simulink model "A_real_IGBT_Model"  (R2017b)
settings: Solver=ode23tb  StartTime=0.0  StopTime=0.01  MaxStep=1e-8  RelTol=1e-8  EnableMultiTasking=on
libraries: powerlib x12, powerlib_extras x2
Description:
  | Copyright 2008-2009 The MathWorks(TM), Inc.
settings Model: ExtModeTrigMode=oneshot  ExtModeArmWhenConnect=off  ExtModeAutoUpdateStatusClock=off  Creator=dkennedy  LastModifiedBy=Crazyyiwen
settings DataIOCC: SaveFormat=Array  SignalLoggingSaveFormat=ModelDataLogs  SignalLoggingName=sigsOut
settings OptimizationCC: BlockReduction=off  BooleanDataType=off  ExpressionDepthLimit=2147483647  InitFltsAndDblsToZero=on  EfficientMapNaN2IntZero=off  LifeSpan=inf
settings DebuggingCC: SaveWithParameterizedLinksMsg=none  UnderspecifiedInitializationDetection=Classic  MergeDetectMultiDrivingBlocksExec=none  SignalResolutionControl=TryResolveAllWithWarning  MultiTaskDSMMsg=warning  FcnCallInpInsideContextMsg=warning  StateNameClashWarn=warning  StrictBusMsg=None  SFUnexpectedBacktrackingDiag=warning  SFNoUnconditionalDefaultTransitionDiag=warning  SFExecutionAtInitializationDiag=none
settings HardwareCC: ProdBitPerPointer=32  ProdBitPerSizeT=32  ProdBitPerPtrDiffT=32  ProdLargestAtomicFloat=None  ProdIntDivRoundTo=Undefined  ProdEndianess=Unspecified  ProdWordSize=32  ProdHWDeviceType=32-bit Generic  TargetBitPerPointer=64  TargetBitPerSizeT=64  TargetBitPerPtrDiffT=64  TargetLongLongMode=on  TargetIntDivRoundTo=Zero  TargetEndianess=LittleEndian  TargetWordSize=64  TargetHWDeviceType=MATLAB Host  ProdEqTarget=off
settings ModelReferenceCC: PropagateSignalLabelsOutOfModel=off
settings RTWCC: Description=Generic Real-Time Target
settings CodeAppCC: StateflowObjectComments=on
settings GRTTargetCC: TargetFcnLib=ansi_tfl_tmw.mat  TargetLangStandard=C89/C90 (ANSI)  GeneratePreprocessorConditionals=Disable all  CombineOutputUpdateFcns=off  GRTInterface=on
settings ConfigComp: CovMetricSettings=dw  CovHtmlReporting=on  CovSaveCumulativeToWorkspaceVar=on  CovSaveSingleToWorkspaceVar=on  CovExternalEMLEnable=off

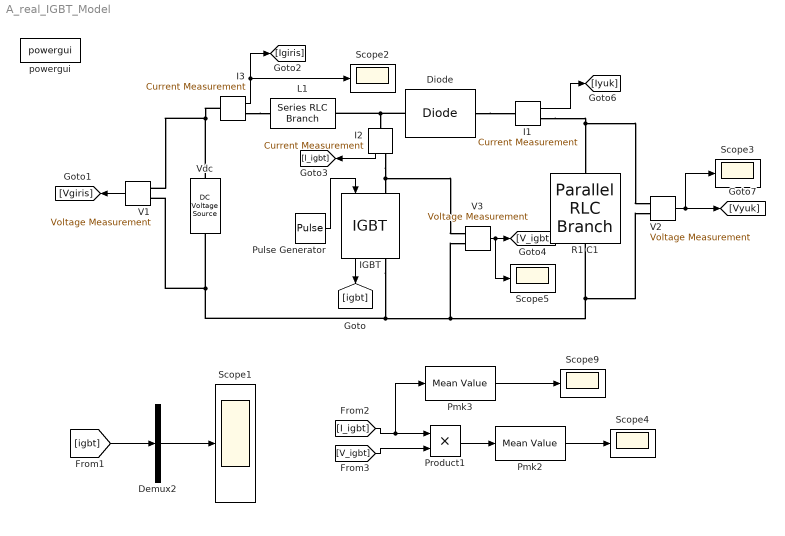
== system A_real_IGBT_Model ==
  " IGBT" : powerlib/Power Electronics/IGBT  Ron=0.01  Lon=0  Vf=1  Tf=1e-6  Tt=1e-6  IC=0  Rs=10000  Cs=inf  Measurements=on
      settings: AttributesFormatString=\n
  Demux2 : Demux  Outputs=1
  Diode : powerlib/Power Electronics/Diode  Ron=0.05  Lon=0  Vf=0.8  IC=0  UseSnubber=off  Rs=1e5  Cs=inf  Measurements=off
  I1 : powerlib/Measurements/Current Measurement  PhasorSimulation=off  OutputType=Complex  PSBequivalent=0
  I2 : powerlib/Measurements/Current Measurement  PhasorSimulation=off  OutputType=Complex  PSBequivalent=0
  I3 : powerlib/Measurements/Current Measurement  PhasorSimulation=off  OutputType=Complex  PSBequivalent=0
  L1 : powerlib/Elements/Series RLC Branch  LConnTagsString=__new0  RConnTagsString=__new0  BranchType=L  Resistance=1.0  Inductance=400e-6  SetiL0=on  InitialCurrent=0  Capacitance=1.0  Setx0=off  InitialVoltage=0  Measurements=Branch current
  Pmk2 : powerlib_extras/Measurements/Mean Value  Period=0.1
  Pmk3 : powerlib_extras/Measurements/Mean Value  Period=0.1
  Product1 : Product  RndMeth=Zero
  Pulse Generator : DiscretePulseGenerator  PulseType=Time based  Amplitude=20  Period=50e-4  PulseWidth=50
  R1 C1 : powerlib/Elements/Parallel RLC Branch  LConnTagsString=a  RConnTagsString=__new0  BranchType=RC  Resistance=50  Inductance=1.0  SetiL0=off  InitialCurrent=0  Capacitance=25e-06  Setx0=on  InitialVoltage=0  Measurements=Branch voltage and current
  Scope{1..5,9} (6 alike) : Scope
  V1 : powerlib/Measurements/Voltage Measurement  PhasorSimulation=off  OutputType=Complex  PSBequivalent=0
  V2 : powerlib/Measurements/Voltage Measurement  PhasorSimulation=off  OutputType=Complex  PSBequivalent=0
  V3 : powerlib/Measurements/Voltage Measurement  PhasorSimulation=off  OutputType=Complex  PSBequivalent=0
  Vdc : powerlib/Electrical Sources/DC Voltage Source  Description=source block  Amplitude=100  Measurements=None
      settings: AttributesFormatString=\n
  powergui : powerlib/powergui  SimulationMode=Continuous  SampleTime=5e-5  frequency=60  Iterations=50  frequencyindice=0  Pbase=100e6  ErrMax=1e-4  UnitsV=kV  UnitsW=MW  buscounter=0  FunctionMessages=off  echomessages=off  EnableUseOfTLC=off  CurrentSourceSwitches=on  DisableSnubberDevices=off  DisableRonSwitches=off  DisableVfSwitches=off  DisplayEquations=off  SolverType=Tustin/Backward Euler (TBE)  Interpol=off  ExternalGateDelay=off  methode=off  Ts=0  x0status=blocks  SPID=off  SwTol=0  HookPort=off  RestoreLinks=warning  ResistiveCurrentMeasurement=off  Frange=[0:2:500]  Ylog=off  Xlog=on  ShowGrid=off  save=off  variable=ZData  structure=0  ZoomFFT=on  StartTime=0.0  cycles=1  DisplayStyle=1  fundamental=60  FreqAxis=off  MaxFrequency=1000  frequencyindicesteady=1  RmsSteady=1  display=off
  wires:
  Pulse Generator/1 -> " IGBT"/1
  " IGBT"/1 -> [igbt]
  [igbt] -> Demux2/1
  Demux2/1 -> Scope1/1
  V1/1 -> [Vgiris]
  I3/1 -> [Igiris], Scope2/1
  I1/1 -> [Iyuk]
  V2/1 -> [Vyuk], Scope3/1
  [I_igbt] -> Product1/1, Pmk3/1
  [V_igbt] -> Product1/2
  I2/1 -> [I_igbt]
  V3/1 -> Scope5/1, [V_igbt]
  Product1/1 -> Pmk2/1
  Pmk2/1 -> Scope4/1
  Pmk3/1 -> Scope9/1
  connections:
  " IGBT"/RConn1 -- Vdc/LConn1 -- V1/LConn2 -- R1 C1/RConn1 -- V2/LConn2 -- V3/LConn2
  I3/LConn1 -- Vdc/RConn1 -- V1/LConn1
  Diode/LConn1 -- L1/RConn1 -- I2/LConn1
  I3/RConn1 -- L1/LConn1
  Diode/RConn1 -- I1/LConn1
  I1/RConn1 -- R1 C1/LConn1 -- V2/LConn1
  I2/RConn1 -- " IGBT"/LConn1 -- V3/LConn1
